simulink model "ParameterEstimation_AkimInputu"  (R2025b)
settings: Solver=ode45  StartTime=0.0  StopTime=60  MaxStep=1e-3  RelTol=1e-3  EnableMultiTasking=on
settings Model: ModifiedByFormat=The MathWorks Inc.  VariantFading=off  Creator=The MathWorks, Inc.  LastModifiedBy=The MathWorks Inc.
settings SolverCC: AlgebraicLoopSolver=TrustRegion
settings DataIOCC: LimitDataPoints=on  SaveFormat=Array  SaveOutput=off  SaveTime=off  ReturnWorkspaceOutputsName=SDOSimTest_Log
settings OptimizationCC: ExpressionDepthLimit=2147483647.0  LifeSpan=1
settings DebuggingCC: UnderspecifiedInitializationDetection=Classic  MergeDetectMultiDrivingBlocksExec=none  SolverPrmCheckMsg=warning  FcnCallInpInsideContextMsg=warning  UnconnectedInputMsg=warning  UnconnectedOutputMsg=warning  UnconnectedLineMsg=warning  StateNameClashWarn=warning  SFUnexpectedBacktrackingDiag=warning  SFNoUnconditionalDefaultTransitionDiag=warning  SFExecutionAtInitializationDiag=none  ArithmeticOperatorsInVariantConditions=warning
settings HardwareCC: ProdBitPerPointer=32.0  ProdBitPerSizeT=32.0  ProdBitPerPtrDiffT=32.0  ProdLargestAtomicFloat=None  ProdIntDivRoundTo=Undefined  ProdEndianess=Unspecified  ProdWordSize=32.0  ProdHWDeviceType=32-bit Generic
settings ModelReferenceCC: PropagateSignalLabelsOutOfModel=off
settings SFSimCC: SimUseLocalCustomCode=off  CustomCodeUndefinedFunction=UseInterfaceOnly
settings RTWCC: RTWUseLocalCustomCode=off  GPUComputeCapability=3.5
settings CodeAppCC: StateflowObjectComments=on
settings GRTTargetCC: TargetLangStandard=C89/C90 (ANSI)  CombineOutputUpdateFcns=off  GRTInterface=on
settings ConfigComp: CovMetricSettings=dw  CovSaveCumulativeToWorkspaceVar=on  CovSaveSingleToWorkspaceVar=on  CovExternalEMLEnable=off  CovSFcnEnable=off

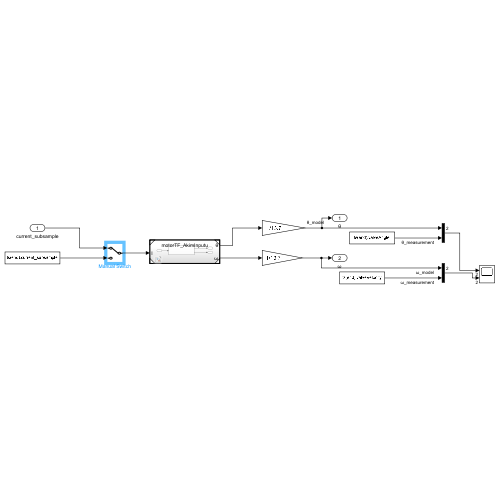
[thumbnail: Simulink's stored preview of the top-level diagram]
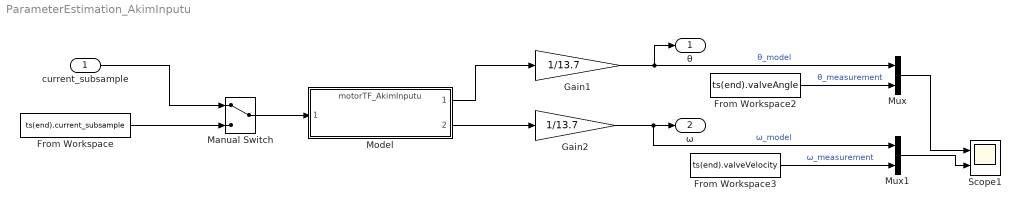
== system ParameterEstimation_AkimInputu ==
  current_subsample : Inport
  From Workspace : FromWorkspace  VariableName=ts(end).current_subsample  SampleTime=1e-3  OutputAfterFinalValue=Setting to zero
  From Workspace2 : FromWorkspace  VariableName=ts(end).valveAngle
  From Workspace3 : FromWorkspace  VariableName=ts(end).valveVelocity
  Gain1 : Gain  Gain=1/13.7
  Gain2 : Gain  Gain=1/13.7
  Manual Switch : ManualSwitch
  Model : ModelReference  ModelNameDialog=motorTF_AkimInputu.slx  SimulationMode=Normal  ModelReferenceVersion=1.5
  Mux : Mux  Inputs=2
  Mux1 : Mux  Inputs=2
  Scope1 : Scope  NumInputPorts=2
      settings: TimeSpan=1  ActiveDisplayYMinimum=-1388.5356702215108  ActiveDisplayYMaximum=6088.3720679833614
  θ : Outport  Unit=deg
  ω : Outport  Port=2  Unit=deg/s
  wires:
  Manual Switch/1 -> Model/1
  current_subsample/1 -> Manual Switch/1
  From Workspace/1 -> Manual Switch/2
  Model/2 -> Gain2/1
  Model/1 -> Gain1/1
  From Workspace2/1 -> Mux/2  "θ_measurement"
  From Workspace3/1 -> Mux1/2  "ω_measurement"
  Gain1/1 -> θ/1, Mux/1  "θ_model"
  Gain2/1 -> Mux1/1, ω/1  "ω_model"
  Mux1/1 -> Scope1/2
  Mux/1 -> Scope1/1
